simulink model "SIH26037_SupervisoryArchitecture"  (R2026a)
settings: Solver=VariableStepAuto
settings Model: Creator=yeswanth  LastModifiedBy=yeswanth

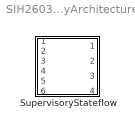
== system SIH26037_SupervisoryArchitecture ==
  SupervisoryStateflow : Stateflow chart  TreatAsAtomicUnit=on

== stateflow chart SIH26037_SupervisoryArchitecture/SupervisoryStateflow ==
  note: SIH26037 HIERARCHICAL STATEFLOW SUPERVISORY ARCHITECTURE
      | Authoritative Stage 5 Execution Model & PPT Reference
  state INIT
    entry:
    macro_intent = uint8(0);
    target_v = 0.0;
    locked_side = uint8(0);
    safety_override = false;
  state AUTONOMOUS_NAVIGATION
    entry:
    safety_override = false;
    state CRUISE
      entry:
      macro_intent = uint8(0);
      target_v = 8.0;
      locked_side = uint8(0);
    state FOLLOW
      entry:
      macro_intent = uint8(1);
      locked_side = uint8(0);
      during:
      target_v = max(0.0, min(8.0, 8.0 + 0.40*(lead_dx - 15.0)));
    state RECOVER
      entry:
      macro_intent = uint8(4);
      locked_side = uint8(0);
      target_v = 8.0;
    state YIELD
      entry:
      macro_intent = uint8(2);
      locked_side = uint8(0);
      during:
      target_v = max(0.0, min(4.0, 0.50*(lead_dx - 15.0)));
    state OVERTAKE
      entry:
      macro_intent = uint8(3);
      locked_side = uint8(1);
      target_v = max(4.0, v_ego + 2.0);
    CRUISE -> FOLLOW [order 1] : [lead_dx <= 40.0 && lead_dx > 28.0]
    YIELD -> FOLLOW [order 2] : [min_ttc > 6.0 && lead_dx > 28.0]
    FOLLOW -> YIELD [order 2] : [min_ttc <= 6.0 || W_avail < 4.10]
    OVERTAKE -> RECOVER [order 1] : [lead_dx >= 7.50]
    CRUISE -> YIELD [order 2] : [min_ttc <= 6.0]
    FOLLOW -> OVERTAKE [order 1] : [lead_dx <= 28.0 && W_avail >= 4.10 && min_ttc > 6.0]
    OVERTAKE -> YIELD [order 2] : [min_ttc <= 6.0]
    YIELD -> OVERTAKE [order 1] : [min_ttc > 6.0 && W_avail >= 4.10 && lead_dx <= 28.0]
  state EMERGENCY
    entry:
    macro_intent = uint8(5);
    target_v = 0.0;
    locked_side = uint8(0);
    safety_override = true;
  state SAFE_STOP
    entry:
    macro_intent = uint8(6);
    target_v = 0.0;
    locked_side = uint8(0);
    safety_override = true;
  state MISSION_COMPLETE
    entry:
    macro_intent = uint8(0);
    target_v = 0.0;
    locked_side = uint8(0);
    safety_override = false;
  (default) -> INIT [order 1]
  (default) -> CRUISE [order 2]
  RECOVER -> CRUISE : [v_ego >= 7.5]
  INIT -> AUTONOMOUS_NAVIGATION : [lead_dx > 0]
  AUTONOMOUS_NAVIGATION -> EMERGENCY : [mpc_status == 0 || min_ttc < 1.0 || clearance <= 0.05]
  EMERGENCY -> SAFE_STOP : [v_ego < 0.10]
  data: lead_dx input double; min_ttc input double; W_avail input double; mpc_status input int32; v_ego input double; clearance input double; macro_intent output uint8; target_v output double; locked_side output uint8; safety_override output boolean
